simulink model "AoA0"  (R2020b)
settings: Solver=ode1  StartTime=0.0  StopTime=.005  FixedStep=.001  RelTol=1e-3
model workspace (MAT data in the model file):
  A = 0.0156
  Cd0p = 0.05
  Cdap = 0.1
  Cl0p = 0.39
  Clap = 4.5
  I3 = 0.0002817
  R = 0.13
  aD = 0.36247
  aDa = 0
  aL = 0.822747
  aLa = 0.253406
  aMx = 0.2663238
  aMxa = 0.119789
  aMy = 0.5
  aMya = 0
  aMz = 0.574602
  aMza = 0.3333333
  bD = 0.272797
  bDa = 0.5
  bL = -0.114013
  bLa = 0.5115438
  bMx = 0.102435
  bMxa = 0.0581454
  bMy = 0
  bMya = 0.5
  bMz = -0.092139
  bMza = 0
  g = 9.81
  m = 0.03
  rho = 1.225
settings Model: Creator=ethan  LastModifiedBy=ethan
settings DataIOCC: SaveOutput=off  SaveTime=off

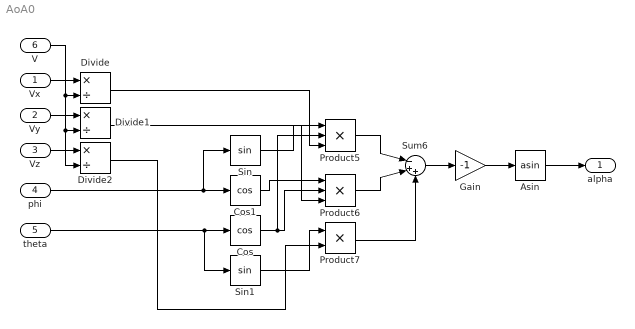
== system AoA0 ==
  Vx : Inport  OutDataTypeStr=double  PortDimensions=1  SampleTime=0
  Vy : Inport  Port=2  OutDataTypeStr=double  PortDimensions=1  SampleTime=0
  Vz : Inport  Port=3  OutDataTypeStr=double  PortDimensions=1  SampleTime=0
  phi : Inport  Port=4  OutDataTypeStr=double  PortDimensions=1  SampleTime=0
  theta : Inport  Port=5  OutDataTypeStr=double  PortDimensions=1  SampleTime=0
  V : Inport  Port=6
  Asin : Trigonometry  Operator=asin
  Cos : Trigonometry  Operator=cos
  Cos1 : Trigonometry  Operator=cos
  Divide : Product  Inputs=*/
  Divide1 : Product  Inputs=*/
  Divide2 : Product  Inputs=*/
  Gain : Gain  Gain=-1
  Product5 : Product  Inputs=3
  Product6 : Product  Inputs=3
  Product7 : Product
  Sin : Trigonometry
  Sin1 : Trigonometry
  Sum6 : Sum  Inputs=|-++
  alpha : Outport  OutDataTypeStr=double  PortDimensions=1  SampleTime=0
  wires:
  Sin/1 -> Product5/1
  Product7/1 -> Sum6/3
  Product6/1 -> Sum6/2
  Product5/1 -> Sum6/1
  Cos/1 -> Product6/2, Product5/2
  Cos1/1 -> Product6/1
  theta/1 -> Sin1/1, Cos/1
  phi/1 -> Cos1/1, Sin/1
  Asin/1 -> alpha/1
  Sin1/1 -> Product7/1
  Vx/1 -> Divide/1
  Vy/1 -> Divide1/1
  Vz/1 -> Divide2/1
  V/1 -> Divide2/2, Divide1/2, Divide/2
  Divide/1 -> Product5/3
  Divide1/1 -> Product6/3
  Divide2/1 -> Product7/2
  Sum6/1 -> Gain/1
  Gain/1 -> Asin/1
